simulink library "Vex_V5_Simulink_Expansion"  (R2022a)
settings: Solver=VariableStepAuto  StartTime=0.0  StopTime=10.0  RelTol=1e-3
libraries: $bdroot x48, vexv5lib x31, dspsigops x6, dsparch4 x2, slpidlib x1
(part 2 of 2)

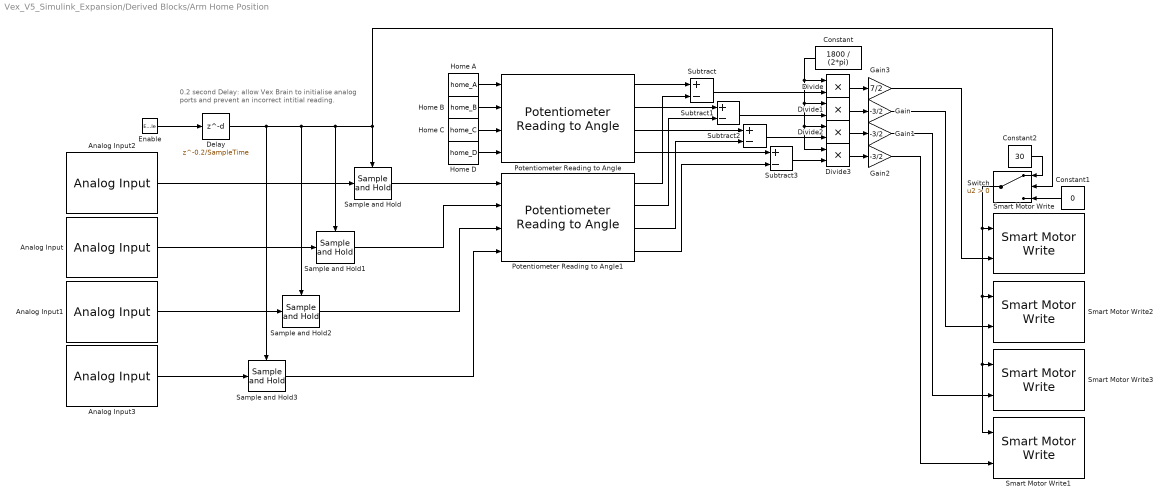
== system Vex_V5_Simulink_Expansion/Derived Blocks/Arm Home Position ==
  note: 0.2 second Delay: allow Vex Brain to initialise
      | analog ports and prevent an incorrect intitial reading.
  Enable : EnablePort  ShowOutputPort=on
  Analog Input : vexv5lib/Sensors/Analog Input  port=B  SampleTime=0.01
      settings: SourceProductBaseCode=VEXV5
  Analog Input1 : vexv5lib/Sensors/Analog Input  port=C  SampleTime=0.01
      settings: SourceProductBaseCode=VEXV5
  Analog Input2 : vexv5lib/Sensors/Analog Input  port=A  SampleTime=0.01
      settings: SourceProductBaseCode=VEXV5
  Analog Input3 : vexv5lib/Sensors/Analog Input  port=D  SampleTime=0.01
      settings: SourceProductBaseCode=VEXV5
  Constant : Constant  Value=1800 / (2*pi)
  Constant1 : Constant  Value=0
  Constant2 : Constant  Value=30
  Delay : Delay  DelayLength=0.2/SampleTime  SampleTime=SampleTime
  Divide{,1..3} (4 alike) : Product  Inputs=**
  Gain : Gain  Gain=-3/2
  Gain1 : Gain  Gain=-3/2
  Gain2 : Gain  Gain=-3/2
  Gain3 : Gain  Gain=7/2
  Home A : Constant  Value=home_A
  Home B : Constant  Value=home_B
  Home C : Constant  Value=home_C
  Home D : Constant  Value=home_D
  Potentiometer Reading to Angle : $bdroot/Unit Conversion/Potentiometer Reading to Angle  Home_A=home_A  Home_B=home_B  Home_C=home_C  Home_D=home_D
  Potentiometer Reading to Angle1 : $bdroot/Unit Conversion/Potentiometer Reading to Angle  Home_A=home_A  Home_B=home_B  Home_C=home_C  Home_D=home_D
  Sample and Hold{,1..3} (4 alike) : dspsigops/Sample and Hold  trig=Rising edge  initCond=0  latchinput=off
  Smart Motor Write : vexv5lib/Actuators/Smart Motor Write  motorPort=1  scaleFactor=18:1  MotorBrakeMode=Coast  OperationMode=Position Control
      settings: SourceProductBaseCode=VEXV5
  Smart Motor Write1 : vexv5lib/Actuators/Smart Motor Write  motorPort=4  scaleFactor=18:1  MotorBrakeMode=Coast  OperationMode=Position Control
      settings: SourceProductBaseCode=VEXV5
  Smart Motor Write2 : vexv5lib/Actuators/Smart Motor Write  motorPort=2  scaleFactor=18:1  MotorBrakeMode=Coast  OperationMode=Position Control
      settings: SourceProductBaseCode=VEXV5
  Smart Motor Write3 : vexv5lib/Actuators/Smart Motor Write  motorPort=3  scaleFactor=18:1  MotorBrakeMode=Coast  OperationMode=Position Control
      settings: SourceProductBaseCode=VEXV5
  Subtract{,1..3} (4 alike) : Sum  Inputs=+-
  Switch : Switch  Criteria=u2 > Threshold  SaturateOnIntegerOverflow=off  InputSameDT=off
  wires:
  Delay/1 -> Sample and Hold3/Trigger, Sample and Hold2/Trigger, Sample and Hold1/Trigger, Switch/2, Sample and Hold/Trigger
  Enable/1 -> Delay/1
  Potentiometer Reading to Angle/4 -> Subtract3/1
  Home C/1 -> Potentiometer Reading to Angle/3
  Gain3/1 -> Smart Motor Write/2
  Gain2/1 -> Smart Motor Write1/2
  Home A/1 -> Potentiometer Reading to Angle/1
  Divide3/1 -> Gain2/1
  Subtract2/1 -> Divide2/2
  Divide/1 -> Gain3/1
  Divide1/1 -> Gain/1
  Subtract/1 -> Divide/2
  Gain/1 -> Smart Motor Write2/2
  Constant1/1 -> Switch/3
  Switch/1 -> Smart Motor Write1/1, Smart Motor Write3/1, Smart Motor Write2/1, Smart Motor Write/1
  Constant2/1 -> Switch/1
  Analog Input1/1 -> Sample and Hold2/1
  Analog Input/1 -> Sample and Hold1/1
  Potentiometer Reading to Angle1/3 -> Subtract2/2
  Subtract1/1 -> Divide1/2
  Analog Input3/1 -> Sample and Hold3/1
  Potentiometer Reading to Angle1/4 -> Subtract3/2
  Gain1/1 -> Smart Motor Write3/2
  Potentiometer Reading to Angle/3 -> Subtract2/1
  Subtract3/1 -> Divide3/2
  Sample and Hold2/1 -> Potentiometer Reading to Angle1/3
  Divide2/1 -> Gain1/1
  Potentiometer Reading to Angle1/2 -> Subtract1/2
  Analog Input2/1 -> Sample and Hold/1
  Sample and Hold3/1 -> Potentiometer Reading to Angle1/4
  Potentiometer Reading to Angle/1 -> Subtract/1
  Constant/1 -> Divide3/1, Divide2/1, Divide1/1, Divide/1
  Sample and Hold/1 -> Potentiometer Reading to Angle1/1
  Potentiometer Reading to Angle/2 -> Subtract1/1
  Home D/1 -> Potentiometer Reading to Angle/4
  Potentiometer Reading to Angle1/1 -> Subtract/2
  Home B/1 -> Potentiometer Reading to Angle/2
  Sample and Hold1/1 -> Potentiometer Reading to Angle1/2

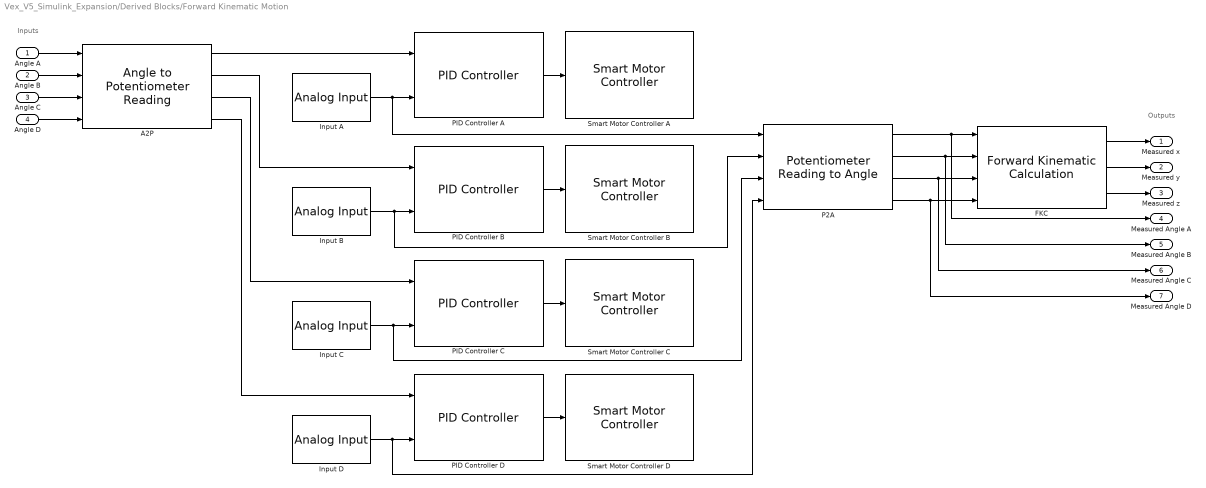
== system Vex_V5_Simulink_Expansion/Derived Blocks/Forward Kinematic Motion ==
  note: Inputs
  note: Outputs
  Angle A : Inport
  Angle B : Inport  Port=2
  Angle C : Inport  Port=3
  Angle D : Inport  Port=4
  A2P : $bdroot/Unit Conversion/Angle to Potentiometer Reading  Home_A=Home_A  Home_B=Home_B  Home_C=Home_C  Home_D=Home_D
  FKC : $bdroot/Core Blocks/Forward Kinematic Calculation
  Input A : vexv5lib/Sensors/Analog Input  port=A  SampleTime=SampleTime
      settings: SourceProductBaseCode=VEXV5
  Input B : vexv5lib/Sensors/Analog Input  port=B  SampleTime=SampleTime
      settings: SourceProductBaseCode=VEXV5
  Input C : vexv5lib/Sensors/Analog Input  port=C  SampleTime=SampleTime
      settings: SourceProductBaseCode=VEXV5
  Input D : vexv5lib/Sensors/Analog Input  port=D  SampleTime=SampleTime
      settings: SourceProductBaseCode=VEXV5
  P2A : $bdroot/Unit Conversion/Potentiometer Reading to Angle  Home_A=Home_A  Home_B=Home_B  Home_C=Home_C  Home_D=Home_D
  PID Controller A : $bdroot/Core Blocks/PID Controller  KP=KP_A  KI=KI_A  KD=KD_A  LimitOutput=off  limitHigh=limitHigh_A  limitLow=limitLow_A  AntiWindupMode=none  kb=kb_A
  PID Controller B : $bdroot/Core Blocks/PID Controller  KP=KP_B  KI=KI_B  KD=KD_B  LimitOutput=off  limitHigh=limitHigh_B  limitLow=limitLow_B  AntiWindupMode=none  kb=kb_B
  PID Controller C : $bdroot/Core Blocks/PID Controller  KP=KP_C  KI=KI_C  KD=KD_C  LimitOutput=off  limitHigh=limitHigh_C  limitLow=limitLow_C  AntiWindupMode=none  kb=kb_C
  PID Controller D : $bdroot/Core Blocks/PID Controller  KP=KP_D  KI=KI_D  KD=KD_D  LimitOutput=off  limitHigh=limitHigh_D  limitLow=limitLow_D  AntiWindupMode=none  kb=kb_D
  Smart Motor Controller A : $bdroot/Core Blocks/Smart Motor Controller  motorPort=1  OperationMode=Advanced Control  MotorBrakeMode=Coast
  Smart Motor Controller B : $bdroot/Core Blocks/Smart Motor Controller  motorPort=2  OperationMode=Advanced Control  MotorBrakeMode=Coast
  Smart Motor Controller C : $bdroot/Core Blocks/Smart Motor Controller  motorPort=3  OperationMode=Advanced Control  MotorBrakeMode=Coast
  Smart Motor Controller D : $bdroot/Core Blocks/Smart Motor Controller  motorPort=4  OperationMode=Advanced Control  MotorBrakeMode=Coast
  Measured x : Outport
  Measured y : Outport  Port=2
  Measured z : Outport  Port=3
  Measured Angle A : Outport  Port=4
  Measured Angle B : Outport  Port=5
  Measured Angle C : Outport  Port=6
  Measured Angle D : Outport  Port=7
  wires:
  A2P/3 -> PID Controller C/1
  PID Controller A/1 -> Smart Motor Controller A/1
  A2P/1 -> PID Controller A/1
  Input C/1 -> PID Controller C/2, P2A/3
  Angle D/1 -> A2P/4
  P2A/4 -> FKC/4, Measured Angle D/1
  P2A/3 -> FKC/3, Measured Angle C/1
  Angle C/1 -> A2P/3
  A2P/4 -> PID Controller D/1
  P2A/2 -> FKC/2, Measured Angle B/1
  FKC/1 -> Measured x/1
  Input B/1 -> PID Controller B/2, P2A/2
  P2A/1 -> FKC/1, Measured Angle A/1
  Input A/1 -> P2A/1, PID Controller A/2
  FKC/3 -> Measured z/1
  Input D/1 -> PID Controller D/2, P2A/4
  FKC/2 -> Measured y/1
  PID Controller B/1 -> Smart Motor Controller B/1
  PID Controller D/1 -> Smart Motor Controller D/1
  Angle A/1 -> A2P/1
  PID Controller C/1 -> Smart Motor Controller C/1
  A2P/2 -> PID Controller B/1
  Angle B/1 -> A2P/2

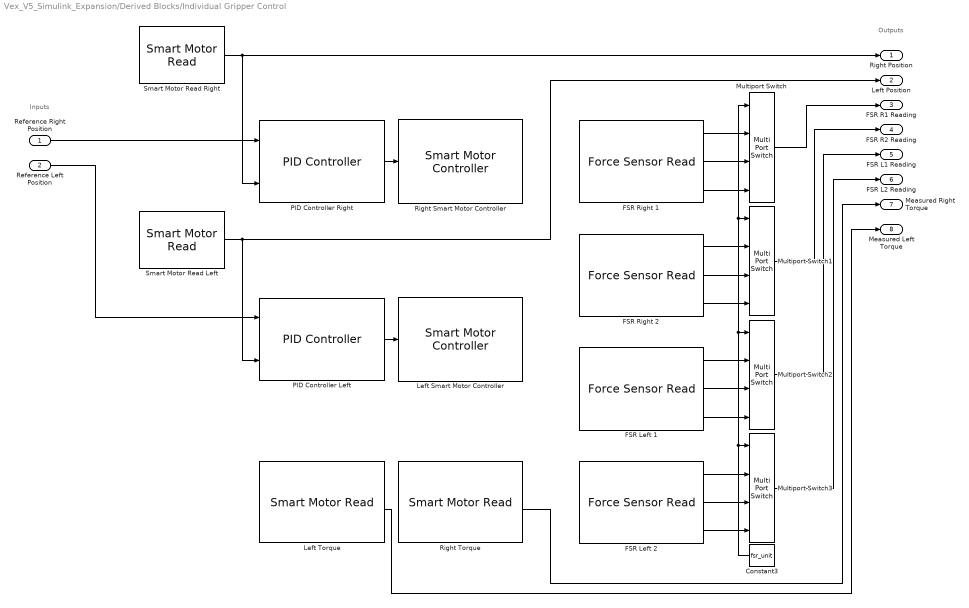
== system Vex_V5_Simulink_Expansion/Derived Blocks/Individual Gripper Control ==
  note: Outputs
  note: Inputs
  Reference Right Position : Inport
  Reference Left Position : Inport  Port=2
  Constant3 : Constant  Value=fsr_unit
  FSR Left 1 : $bdroot/Core Blocks/Force Sensor Read  port=A  SampleTime=SampleTime  Value=LA
  FSR Left 2 : $bdroot/Core Blocks/Force Sensor Read  port=B  SampleTime=SampleTime  Value=LB
  FSR Right 1 : $bdroot/Core Blocks/Force Sensor Read  port=D  SampleTime=SampleTime  Value=RA
  FSR Right 2 : $bdroot/Core Blocks/Force Sensor Read  port=C  SampleTime=SampleTime  Value=RB
  Left Smart Motor Controller : $bdroot/Core Blocks/Smart Motor Controller  motorPort=6  OperationMode=Advanced Control  MotorBrakeMode=Coast
  Left Torque : $bdroot/Core Blocks/Smart Motor Read  motorPort=6  SampleTime=SampleTime
  Multiport Switch{,1..3} (4 alike) : MultiPortSwitch  SaturateOnIntegerOverflow=off  InputSameDT=off
  PID Controller Left : $bdroot/Core Blocks/PID Controller  KP=KP  KI=KI  KD=KD  LimitOutput=off  limitHigh=limitHigh  limitLow=limitLow  AntiWindupMode=none  kb=kb
  PID Controller Right : $bdroot/Core Blocks/PID Controller  KP=KP  KI=KI  KD=KD  LimitOutput=off  limitHigh=limitHigh  limitLow=limitLow  AntiWindupMode=none  kb=kb
  Right Smart Motor Controller : $bdroot/Core Blocks/Smart Motor Controller  motorPort=3  OperationMode=Advanced Control  MotorBrakeMode=Coast
  Right Torque : $bdroot/Core Blocks/Smart Motor Read  motorPort=3  SampleTime=SampleTime
  Smart Motor Read Left : vexv5lib/Sensors/Smart Motor Read  motorPort=6  EncoderUnit=Degrees  resetOption=No reset  additionalOutput=off  SampleTime=SampleTime
      settings: SourceProductBaseCode=VEXV5
  Smart Motor Read Right : vexv5lib/Sensors/Smart Motor Read  motorPort=3  EncoderUnit=Degrees  resetOption=No reset  additionalOutput=off  SampleTime=SampleTime
      settings: SourceProductBaseCode=VEXV5
  Right Position : Outport
  Left Position : Outport  Port=2
  FSR R1 Reading : Outport  Port=3
  FSR R2 Reading : Outport  Port=4
  FSR L1 Reading : Outport  Port=5
  FSR L2 Reading : Outport  Port=6
  Measured Right Torque : Outport  Port=7
  Measured Left Torque : Outport  Port=8
  wires:
  Reference Right Position/1 -> PID Controller Right/1
  Reference Left Position/1 -> PID Controller Left/1
  FSR Right 1/1 -> Multiport Switch/2
  FSR Right 1/2 -> Multiport Switch/3
  FSR Right 1/3 -> Multiport Switch/4
  FSR Right 2/1 -> Multiport Switch1/2
  FSR Right 2/2 -> Multiport Switch1/3
  FSR Right 2/3 -> Multiport Switch1/4
  FSR Left 1/1 -> Multiport Switch2/2
  FSR Left 1/2 -> Multiport Switch2/3
  FSR Left 1/3 -> Multiport Switch2/4
  FSR Left 2/1 -> Multiport Switch3/2
  FSR Left 2/2 -> Multiport Switch3/3
  FSR Left 2/3 -> Multiport Switch3/4
  Multiport Switch/1 -> FSR R1 Reading/1
  Multiport Switch1/1 -> FSR R2 Reading/1
  Multiport Switch2/1 -> FSR L1 Reading/1
  Multiport Switch3/1 -> FSR L2 Reading/1
  Constant3/1 -> Multiport Switch/1, Multiport Switch1/1, Multiport Switch2/1, Multiport Switch3/1
  Smart Motor Read Right/1 -> Right Position/1, PID Controller Right/2
  Smart Motor Read Left/1 -> Left Position/1, PID Controller Left/2
  PID Controller Right/1 -> Right Smart Motor Controller/1
  PID Controller Left/1 -> Left Smart Motor Controller/1
  Right Torque/4 -> Measured Right Torque/1
  Left Torque/4 -> Measured Left Torque/1

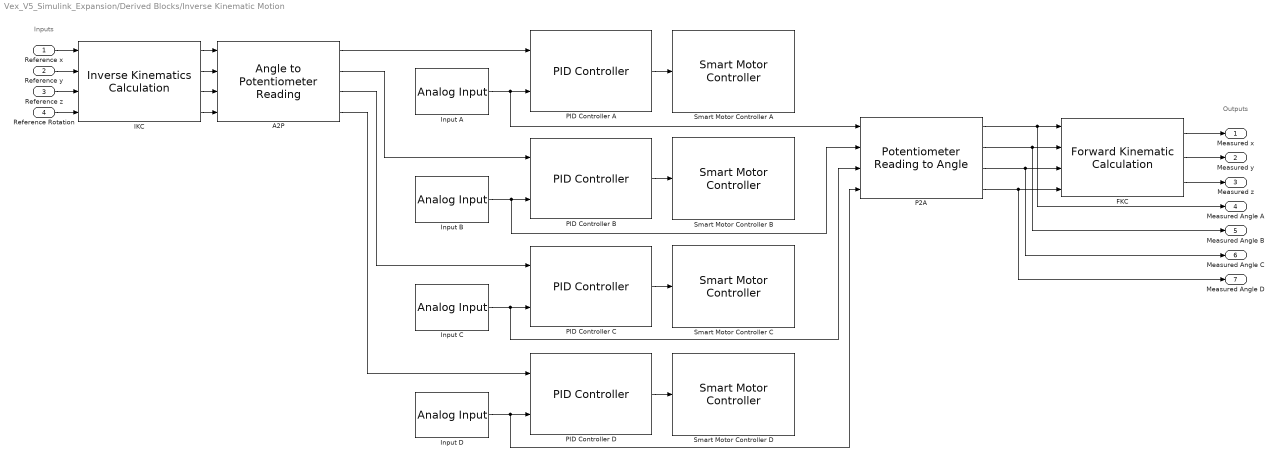
== system Vex_V5_Simulink_Expansion/Derived Blocks/Inverse Kinematic Motion ==
  note: Outputs
  note: Inputs
  Reference x : Inport
  Reference y : Inport  Port=2
  Reference z : Inport  Port=3
  Reference Rotation : Inport  Port=4
  A2P : $bdroot/Unit Conversion/Angle to Potentiometer Reading  Home_A=Home_A  Home_B=Home_B  Home_C=Home_C  Home_D=Home_D
  FKC : $bdroot/Core Blocks/Forward Kinematic Calculation
  IKC : $bdroot/Core Blocks/Inverse Kinematics Calculation
  Input A : vexv5lib/Sensors/Analog Input  port=A  SampleTime=0.01
      settings: SourceProductBaseCode=VEXV5
  Input B : vexv5lib/Sensors/Analog Input  port=B  SampleTime=0.01
      settings: SourceProductBaseCode=VEXV5
  Input C : vexv5lib/Sensors/Analog Input  port=C  SampleTime=0.01
      settings: SourceProductBaseCode=VEXV5
  Input D : vexv5lib/Sensors/Analog Input  port=D  SampleTime=0.01
      settings: SourceProductBaseCode=VEXV5
  P2A : $bdroot/Unit Conversion/Potentiometer Reading to Angle  Home_A=Home_A  Home_B=Home_B  Home_C=Home_C  Home_D=Home_D
  PID Controller A : $bdroot/Core Blocks/PID Controller  KP=KP_A  KI=KI_A  KD=KD_A  LimitOutput=off  limitHigh=limitHigh_A  limitLow=limitLow_A  AntiWindupMode=none  kb=kb_A
  PID Controller B : $bdroot/Core Blocks/PID Controller  KP=KP_B  KI=KI_B  KD=KD_B  LimitOutput=off  limitHigh=limitHigh_B  limitLow=limitLow_B  AntiWindupMode=none  kb=kb_B
  PID Controller C : $bdroot/Core Blocks/PID Controller  KP=KP_C  KI=KI_C  KD=KD_C  LimitOutput=off  limitHigh=limitHigh_C  limitLow=limitLow_C  AntiWindupMode=none  kb=kb_C
  PID Controller D : $bdroot/Core Blocks/PID Controller  KP=KP_D  KI=KI_D  KD=KD_D  LimitOutput=off  limitHigh=limitHigh_D  limitLow=limitLow_D  AntiWindupMode=none  kb=kb_D
  Smart Motor Controller A : $bdroot/Core Blocks/Smart Motor Controller  motorPort=1  OperationMode=Advanced Control  MotorBrakeMode=Coast
  Smart Motor Controller B : $bdroot/Core Blocks/Smart Motor Controller  motorPort=2  OperationMode=Advanced Control  MotorBrakeMode=Coast
  Smart Motor Controller C : $bdroot/Core Blocks/Smart Motor Controller  motorPort=3  OperationMode=Advanced Control  MotorBrakeMode=Coast
  Smart Motor Controller D : $bdroot/Core Blocks/Smart Motor Controller  motorPort=4  OperationMode=Advanced Control  MotorBrakeMode=Coast
  Measured x : Outport
  Measured y : Outport  Port=2
  Measured z : Outport  Port=3
  Measured Angle A : Outport  Port=4
  Measured Angle B : Outport  Port=5
  Measured Angle C : Outport  Port=6
  Measured Angle D : Outport  Port=7
  wires:
  A2P/2 -> PID Controller B/1
  FKC/2 -> Measured y/1
  Input C/1 -> PID Controller C/2, P2A/3
  PID Controller C/1 -> Smart Motor Controller C/1
  Input A/1 -> P2A/1, PID Controller A/2
  PID Controller A/1 -> Smart Motor Controller A/1
  PID Controller B/1 -> Smart Motor Controller B/1
  PID Controller D/1 -> Smart Motor Controller D/1
  FKC/3 -> Measured z/1
  P2A/1 -> FKC/1, Measured Angle A/1
  A2P/1 -> PID Controller A/1
  A2P/4 -> PID Controller D/1
  Input B/1 -> PID Controller B/2, P2A/2
  P2A/3 -> FKC/3, Measured Angle C/1
  Input D/1 -> PID Controller D/2, P2A/4
  FKC/1 -> Measured x/1
  P2A/2 -> FKC/2, Measured Angle B/1
  P2A/4 -> FKC/4, Measured Angle D/1
  IKC/1 -> A2P/1
  IKC/2 -> A2P/2
  IKC/3 -> A2P/3
  IKC/4 -> A2P/4
  Reference x/1 -> IKC/1
  Reference y/1 -> IKC/2
  Reference z/1 -> IKC/3
  Reference Rotation/1 -> IKC/4
  A2P/3 -> PID Controller C/1

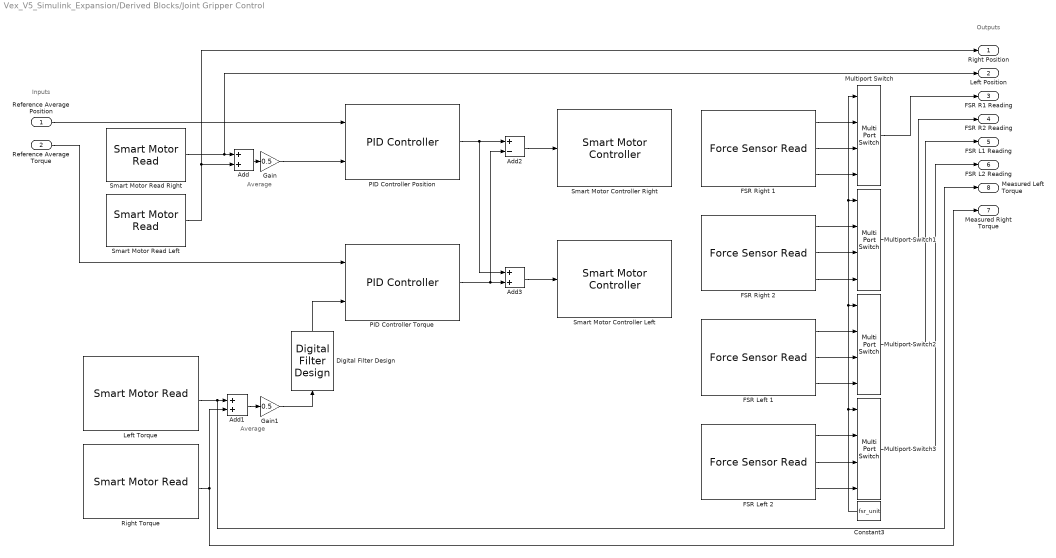
== system Vex_V5_Simulink_Expansion/Derived Blocks/Joint Gripper Control ==
  note: Average
  note: Inputs
  note: Outputs
  note: Average
  Reference Average Position : Inport
  Reference Average Torque : Inport  Port=2
  Add : Sum
  Add1 : Sum
  Add2 : Sum  Inputs=+-
  Add3 : Sum
  Constant3 : Constant  Value=fsr_unit
  Digital Filter Design : dsparch4/Digital Filter Design  mwdsp_browser_bugfix_var=off
  FSR Left 1 : $bdroot/Core Blocks/Force Sensor Read  port=H  SampleTime=SampleTime  Value=LA
  FSR Left 2 : $bdroot/Core Blocks/Force Sensor Read  port=G  SampleTime=SampleTime  Value=LB
  FSR Right 1 : $bdroot/Core Blocks/Force Sensor Read  port=F  SampleTime=SampleTime  Value=RA
  FSR Right 2 : $bdroot/Core Blocks/Force Sensor Read  port=E  SampleTime=SampleTime  Value=RB
  Gain : Gain  Gain=0.5
  Gain1 : Gain  Gain=0.5
  Left Torque : $bdroot/Core Blocks/Smart Motor Read  motorPort=5  SampleTime=SampleTime
  Multiport Switch{,1..3} (4 alike) : MultiPortSwitch  SaturateOnIntegerOverflow=off  InputSameDT=off
  PID Controller Position : $bdroot/Core Blocks/PID Controller  KP=KP_position  KI=KI_positon  KD=KD_position  LimitOutput=off  limitHigh=limitHigh_position  limitLow=limitLow_position  AntiWindupMode=none  kb=kb_position
  PID Controller Torque : $bdroot/Core Blocks/PID Controller  KP=KP  KI=KI  KD=KD  LimitOutput=off  limitHigh=limitHigh  limitLow=limitLow  AntiWindupMode=none  kb=kb
  Right Torque : $bdroot/Core Blocks/Smart Motor Read  motorPort=6  SampleTime=SampleTime
  Smart Motor Controller Left : $bdroot/Core Blocks/Smart Motor Controller  motorPort=5  OperationMode=Advanced Control  MotorBrakeMode=Coast
  Smart Motor Controller Right : $bdroot/Core Blocks/Smart Motor Controller  motorPort=6  OperationMode=Advanced Control  MotorBrakeMode=Coast
  Smart Motor Read Left : vexv5lib/Sensors/Smart Motor Read  motorPort=5  EncoderUnit=Degrees  resetOption=No reset  additionalOutput=off  SampleTime=SampleTime
      settings: SourceProductBaseCode=VEXV5
  Smart Motor Read Right : vexv5lib/Sensors/Smart Motor Read  motorPort=6  EncoderUnit=Degrees  resetOption=No reset  additionalOutput=off  SampleTime=SampleTime
      settings: SourceProductBaseCode=VEXV5
  Right Position : Outport
  Left Position : Outport  Port=2
  FSR R1 Reading : Outport  Port=3
  FSR R2 Reading : Outport  Port=4
  FSR L1 Reading : Outport  Port=5
  FSR L2 Reading : Outport  Port=6
  Measured Right Torque : Outport  Port=7
  Measured Left Torque : Outport  Port=8
  wires:
  FSR Right 2/1 -> Multiport Switch1/2
  FSR Right 2/3 -> Multiport Switch1/4
  FSR Left 1/1 -> Multiport Switch2/2
  FSR Right 1/2 -> Multiport Switch/3
  Reference Average Torque/1 -> PID Controller Torque/1
  Constant3/1 -> Multiport Switch/1, Multiport Switch1/1, Multiport Switch2/1, Multiport Switch3/1
  Multiport Switch3/1 -> FSR L2 Reading/1
  FSR Left 1/2 -> Multiport Switch2/3
  FSR Left 2/3 -> Multiport Switch3/4
  FSR Right 2/2 -> Multiport Switch1/3
  Multiport Switch1/1 -> FSR R2 Reading/1
  FSR Right 1/3 -> Multiport Switch/4
  FSR Left 2/1 -> Multiport Switch3/2
  FSR Left 2/2 -> Multiport Switch3/3
  Multiport Switch/1 -> FSR R1 Reading/1
  FSR Right 1/1 -> Multiport Switch/2
  Multiport Switch2/1 -> FSR L1 Reading/1
  FSR Left 1/3 -> Multiport Switch2/4
  Reference Average Position/1 -> PID Controller Position/1
  Smart Motor Read Right/1 -> Left Position/1, Add/1
  Smart Motor Read Left/1 -> Add/2, Right Position/1
  Add/1 -> Gain/1
  Gain/1 -> PID Controller Position/2
  Add1/1 -> Gain1/1
  Left Torque/4 -> Measured Left Torque/1, Add1/1
  Right Torque/4 -> Measured Right Torque/1, Add1/2
  PID Controller Torque/1 -> Add2/2, Add3/2
  Gain1/1 -> Digital Filter Design/1
  PID Controller Position/1 -> Add3/1, Add2/1
  Add2/1 -> Smart Motor Controller Right/1
  Add3/1 -> Smart Motor Controller Left/1
  Digital Filter Design/1 -> PID Controller Torque/2

== system Vex_V5_Simulink_Expansion/Derived Blocks/Motor Torque Control ==
  note: Outputs
  note: Inputs
  Reference Torque : Inport
  Digital Filter Design : dsparch4/Digital Filter Design  mwdsp_browser_bugfix_var=off
  Motor Read : $bdroot/Core Blocks/Smart Motor Read  motorPort=5  SampleTime=SampleTime
  PID : $bdroot/Core Blocks/PID Controller  KP=KP  KI=KI  KD=KD  LimitOutput=off  limitHigh=limitHigh  limitLow=limitLow  AntiWindupMode=none  kb=kb
  Smart Motor Controller : $bdroot/Core Blocks/Smart Motor Controller  motorPort=5  OperationMode=Advanced Control  MotorBrakeMode=Coast
  Measured Torque : Outport
  Measured Voltage : Outport  Port=2
  Measured Current : Outport  Port=3
  wires:
  Reference Torque/1 -> PID/1
  PID/1 -> Smart Motor Controller/1
  Motor Read/1 -> Measured Voltage/1
  Motor Read/2 -> Measured Current/1
  Motor Read/4 -> Digital Filter Design/1
  Digital Filter Design/1 -> PID/2, Measured Torque/1

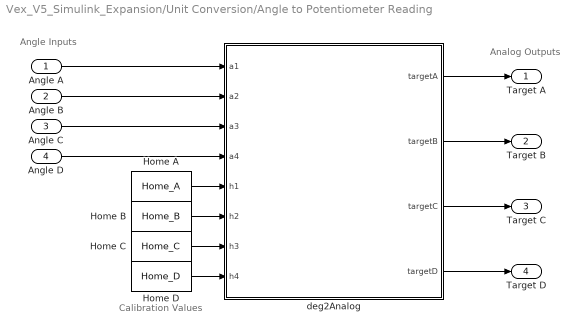
== system Vex_V5_Simulink_Expansion/Unit Conversion/Angle to Potentiometer Reading ==
  note: Calibration Values
  note: Angle Inputs
  note: Analog Outputs
  Angle A : Inport
  Angle B : Inport  Port=2
  Angle C : Inport  Port=3
  Angle D : Inport  Port=4
  Home A : Constant  Value=Home_A
  Home B : Constant  Value=Home_B
  Home C : Constant  Value=Home_C
  Home D : Constant  Value=Home_D
  deg2Analog : MATLAB Function  TreatAsAtomicUnit=on
  Target A : Outport
  Target B : Outport  Port=2
  Target C : Outport  Port=3
  Target D : Outport  Port=4
  wires:
  Home A/1 -> deg2Analog/5(h1)
  Home B/1 -> deg2Analog/6(h2)
  Home C/1 -> deg2Analog/7(h3)
  Home D/1 -> deg2Analog/8(h4)
  Angle D/1 -> deg2Analog/4(a4)
  Angle C/1 -> deg2Analog/3(a3)
  Angle B/1 -> deg2Analog/2(a2)
  Angle A/1 -> deg2Analog/1(a1)
  deg2Analog/1(targetA) -> Target A/1
  deg2Analog/2(targetB) -> Target B/1
  deg2Analog/3(targetC) -> Target C/1
  deg2Analog/4(targetD) -> Target D/1

== system Vex_V5_Simulink_Expansion/Unit Conversion/Force to Resistance ==
  note: Input
  note: Output
  Force : Inport
  Constant : Constant  Value=K
  Constant1 : Constant
  Divide : Product  Inputs=*/
  Divide1 : Product  Inputs=*/
  Gradient : Constant  Value=m
  Power : Math  Operator=pow
  Resistance : Outport
  wires:
  Power/1 -> Resistance/1
  Force/1 -> Divide/1
  Constant/1 -> Divide/2
  Gradient/1 -> Divide1/2
  Constant1/1 -> Divide1/1
  Divide/1 -> Power/1
  Divide1/1 -> Power/2

== system Vex_V5_Simulink_Expansion/Unit Conversion/Joint to Motor Angle ==
  note: Outputs
  note: Inputs
  Joint Angle A : Inport
  Joint Angle B : Inport  Port=2
  Joint Angle C : Inport  Port=3
  Joint Angle D : Inport  Port=4
  jointToMotor : MATLAB Function  TreatAsAtomicUnit=on
  Motor Angle A : Outport
  Motor Angle B : Outport  Port=2
  Motor Angle C : Outport  Port=3
  Motor Angle D : Outport  Port=4
  wires:
  jointToMotor/1(motorA) -> Motor Angle A/1
  jointToMotor/2(motorB) -> Motor Angle B/1
  jointToMotor/3(motorC) -> Motor Angle C/1
  jointToMotor/4(motorD) -> Motor Angle D/1
  Joint Angle D/1 -> jointToMotor/4(jointD)
  Joint Angle C/1 -> jointToMotor/3(jointC)
  Joint Angle B/1 -> jointToMotor/2(jointB)
  Joint Angle A/1 -> jointToMotor/1(jointA)

== system Vex_V5_Simulink_Expansion/Unit Conversion/Motor to Joint Angle ==
  note: Inputs
  note: Outputs
  Motor Angle A : Inport
  Motor Angle B : Inport  Port=2
  Motor Angle C : Inport  Port=3
  Motor Angle D : Inport  Port=4
  motorToJoint : MATLAB Function  TreatAsAtomicUnit=on
  Joint Angle A : Outport
  Joint Angle B : Outport  Port=2
  Joint Angle C : Outport  Port=3
  Joint Angle D : Outport  Port=4
  wires:
  Motor Angle A/1 -> motorToJoint/1(motorA)
  Motor Angle B/1 -> motorToJoint/2(motorB)
  Motor Angle C/1 -> motorToJoint/3(motorC)
  Motor Angle D/1 -> motorToJoint/4(motorD)
  motorToJoint/4(jointD) -> Joint Angle D/1
  motorToJoint/3(jointC) -> Joint Angle C/1
  motorToJoint/2(jointB) -> Joint Angle B/1
  motorToJoint/1(jointA) -> Joint Angle A/1

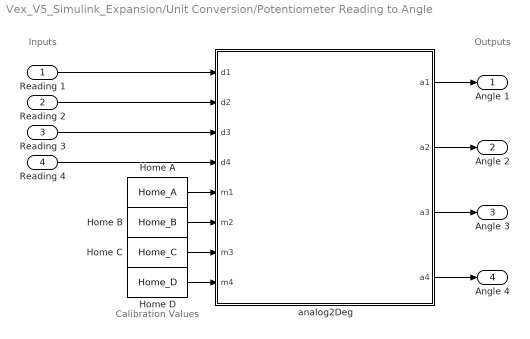
== system Vex_V5_Simulink_Expansion/Unit Conversion/Potentiometer Reading to Angle ==
  note: Outputs
  note: Inputs
  note: Calibration Values
  Reading 1 : Inport
  Reading 2 : Inport  Port=2
  Reading 3 : Inport  Port=3
  Reading 4 : Inport  Port=4
  Home A : Constant  Value=Home_A
  Home B : Constant  Value=Home_B
  Home C : Constant  Value=Home_C
  Home D : Constant  Value=Home_D
  analog2Deg : MATLAB Function  TreatAsAtomicUnit=on
  Angle 1 : Outport
  Angle 2 : Outport  Port=2
  Angle 3 : Outport  Port=3
  Angle 4 : Outport  Port=4
  wires:
  analog2Deg/1(a1) -> Angle 1/1
  analog2Deg/2(a2) -> Angle 2/1
  analog2Deg/3(a3) -> Angle 3/1
  analog2Deg/4(a4) -> Angle 4/1
  Reading 1/1 -> analog2Deg/1(d1)
  Reading 2/1 -> analog2Deg/2(d2)
  Reading 3/1 -> analog2Deg/3(d3)
  Reading 4/1 -> analog2Deg/4(d4)
  Home A/1 -> analog2Deg/5(m1)
  Home B/1 -> analog2Deg/6(m2)
  Home C/1 -> analog2Deg/7(m3)
  Home D/1 -> analog2Deg/8(m4)

== system Vex_V5_Simulink_Expansion/Unit Conversion/Resistance to Force ==
  note: Output
  note: Input
  Resistance : Inport
  Constant : Constant  Value=K
  Divide : Product  Inputs=**
  Gradient : Constant  Value=m
  Power : Math  Operator=pow
  Force : Outport
  wires:
  Gradient/1 -> Power/2
  Power/1 -> Divide/2
  Constant/1 -> Divide/1
  Resistance/1 -> Power/1
  Divide/1 -> Force/1

== system Vex_V5_Simulink_Expansion/Unit Conversion/deg2Rad ==
  Input : Inport
  Constant : Constant  Value=pi
  Constant1 : Constant  Value=180
  Divide : Product  Inputs=**/
  Output : Outport
  wires:
  Input/1 -> Divide/2
  Divide/1 -> Output/1
  Constant/1 -> Divide/1
  Constant1/1 -> Divide/3

== system Vex_V5_Simulink_Expansion/Unit Conversion/rad2Deg ==
  Input : Inport
  Constant : Constant  Value=180
  Constant1 : Constant  Value=pi
  Divide : Product  Inputs=**/
  Output : Outport
  wires:
  Constant1/1 -> Divide/3
  Constant/1 -> Divide/1
  Divide/1 -> Output/1
  Input/1 -> Divide/2

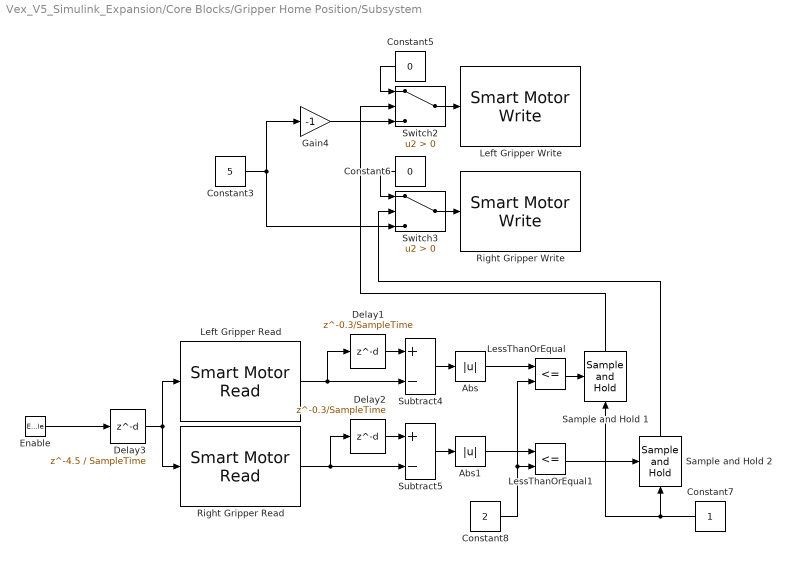
== system Vex_V5_Simulink_Expansion/Core Blocks/Gripper Home Position/Subsystem ==
  Enable : EnablePort  ShowOutputPort=on
  Abs : Abs  SaturateOnIntegerOverflow=off
  Abs1 : Abs  SaturateOnIntegerOverflow=off
  Constant3 : Constant  Value=5
  Constant5 : Constant  Value=0
  Constant6 : Constant  Value=0
  Constant7 : Constant
  Constant8 : Constant  Value=2
  Delay1 : Delay  DelayLength=0.3/SampleTime  SampleTime=SampleTime
  Delay2 : Delay  DelayLength=0.3/SampleTime  SampleTime=SampleTime
  Delay3 : Delay  DelayLength=4.5 / SampleTime  SampleTime=SampleTime
  Gain4 : Gain  Gain=-1
  Left Gripper Read : vexv5lib/Sensors/Smart Motor Read  motorPort=5  EncoderUnit=Degrees  resetOption=Reset by external signal  additionalOutput=off  SampleTime=SampleTime
      settings: SourceProductBaseCode=VEXV5
  Left Gripper Write : vexv5lib/Actuators/Smart Motor Write  motorPort=5  scaleFactor=18:1  MotorBrakeMode=Coast  OperationMode=Velocity Control
      settings: SourceProductBaseCode=VEXV5
  LessThanOrEqual : RelationalOperator  Operator=<=  OutDataTypeStr=boolean  RndMeth=Simplest  InputSameDT=off
  LessThanOrEqual1 : RelationalOperator  Operator=<=  OutDataTypeStr=boolean  RndMeth=Simplest  InputSameDT=off
  Right Gripper Read : vexv5lib/Sensors/Smart Motor Read  motorPort=6  EncoderUnit=Degrees  resetOption=Reset by external signal  additionalOutput=off  SampleTime=SampleTime
      settings: SourceProductBaseCode=VEXV5
  Right Gripper Write : vexv5lib/Actuators/Smart Motor Write  motorPort=6  scaleFactor=18:1  MotorBrakeMode=Coast  OperationMode=Velocity Control
      settings: SourceProductBaseCode=VEXV5
  Sample and Hold 1 : dspsigops/Sample and Hold  trig=Rising edge  initCond=0  latchinput=off
  Sample and Hold 2 : dspsigops/Sample and Hold  trig=Rising edge  initCond=0  latchinput=off
  Subtract4 : Sum  Inputs=+-
  Subtract5 : Sum  Inputs=+-
  Switch2 : Switch  Criteria=u2 > Threshold  SaturateOnIntegerOverflow=off  InputSameDT=off
  Switch3 : Switch  Criteria=u2 > Threshold  SaturateOnIntegerOverflow=off  InputSameDT=off
  wires:
  Switch2/1 -> Left Gripper Write/1
  Constant8/1 -> LessThanOrEqual/2, LessThanOrEqual1/2
  Constant6/1 -> Switch3/1
  Constant7/1 -> Sample and Hold 1/1, Sample and Hold 2/1
  Subtract4/1 -> Abs/1
  Constant5/1 -> Switch2/1
  Delay3/1 -> Left Gripper Read/1, Right Gripper Read/1
  Left Gripper Read/1 -> Delay1/1, Subtract4/2
  Switch3/1 -> Right Gripper Write/1
  LessThanOrEqual/1 -> Sample and Hold 1/Trigger
  Gain4/1 -> Switch2/3
  Right Gripper Read/1 -> Delay2/1, Subtract5/2
  Abs1/1 -> LessThanOrEqual1/1
  Constant3/1 -> Gain4/1, Switch3/3
  Delay2/1 -> Subtract5/1
  Sample and Hold 1/1 -> Switch2/2
  LessThanOrEqual1/1 -> Sample and Hold 2/Trigger
  Abs/1 -> LessThanOrEqual/1
  Enable/1 -> Delay3/1
  Delay1/1 -> Subtract4/1
  Subtract5/1 -> Abs1/1
  Sample and Hold 2/1 -> Switch3/2

== stateflow chart Vex_V5_Simulink_Expansion/Core Blocks/Initialisation Routine/Initialisation Schedule ==
  state Homing
    enable_homing = 1;
    enable_user = 0;
  state User
    enable_homing = 0;
    enable_user = 1;
  (default) -> Homing
  Homing -> User : [simulation_time > 5]
  data: simulation_time input; enable_homing output; enable_user output

== matlab function Vex_V5_Simulink_Expansion/Unit Conversion/Potentiometer Reading to Angle/analog2Deg ==
  data: d1 input; d2 input; d3 input; d4 input; a1 output; m1 input; m2 input; m3 input; m4 input; a2 output; a3 output; a4 output
function [a1,a2,a3,a4] = analog2Deg(d1,d2,d3,d4,m1,m2,m3,m4)
    
    % Vex Brain has a 10 bit ADC == 4096 resolution
    % Potentiometer has 333 degrees of rotation
    scale = ((4096 / 333)*360) / (2*pi);

    % Home angles
    conv = 2*pi / 360;
    ang1 = 0;
    ang2 = 20*conv;
    ang3 = 3.07*conv;
    ang4 = 93.07*conv;

    % Find angles relative to home position
    t1 = (d1 - m1) / scale;
    t2 = (m2 - d2) / (3*scale);
    t3 = (m3 - d3) / (3*scale);
    t4 = (m4 - d4) / (3*scale);

    % Compute actual motor angles
    a1 = t1 + ang1;
    a2 = t2 + ang2;
    a3 = t3 + ang3;
    a4 = t4 + ang4;

== matlab function Vex_V5_Simulink_Expansion/Core Blocks/Force Sensor Read/MATLAB Function ==
  data: volIn input; volOut input; res input; forceRes output
function forceRes = invPD(volIn,volOut,res)
    forceRes = (volIn / volOut)*res - res;

== matlab function Vex_V5_Simulink_Expansion/Core Blocks/Inverse Kinematics Calculation/MATLAB Function ==
  data: x input; a1 output; y input; z input; rotation input; a2 output; a3 output; a4 output
function [a1,a2,a3,a4]= inverseKinematics(x,y,z,rotation)

    % Geometric constants
    conv = 25.4;
    L_1 = 7*conv;
    L_2 = 7*conv;
    L_3 = 2*conv;
    AR = 0.7224*conv;
    AZ = (5.296+1.375)*conv;

    % Handle end effector position/rotation
    x_adj = x - L_3*sin(rotation)*cos(atan(y/x));
    y_adj = y - L_3*sin(rotation)*sin(atan(y/x));
    z_adj = z - L_3*cos(rotation);
    t4 = rotation;

    % Fix base angle to reduce unknowns
    t1 = atan(y_adj/x_adj);
    XE = sqrt(x_adj^2 + y_adj^2) - AR;
    YE = z_adj - AZ;
    
    % Derived using Matlab Symbolic Maths
    t2 = 2*atan((2*L_1*XE - (- L_1^4 + 2*L_1^2*L_2^2 + 2*L_1^2*XE^2 + ...
        2*L_1^2*YE^2 - L_2^4 + 2*L_2^2*XE^2 + 2*L_2^2*YE^2 - XE^4 - ...
        2*XE^2*YE^2 - YE^4)^(1/2))/(L_1^2 + 2*L_1*YE - L_2^2 + XE^2 + YE^2));
    
    % As above
    t3 = 2*atan((2*L_2*XE - ((- L_1^2 + 2*L_1*L_2 - L_2^2 + XE^2 + YE^2) ...
        *(L_1^2 + 2*L_1*L_2 + L_2^2 - XE^2 - YE^2))^(1/2))/ ...
        (- L_1^2 + L_2^2 - 2*L_2*YE + XE^2 + YE^2));

    % Above formulas can produce complex results, the following fixes that
    a1 = NaN(size(t1));
    a2 = NaN(size(t2));
    a3 = NaN(size(t3));
    a4 = NaN(size(t4));

    tf_mat = imag(t1) == 0;
    a1(tf_mat) = real(t1(tf_mat));

    tf_mat = imag(t2) == 0;
    a2(tf_mat) = real(t2(tf_mat));

    tf_mat = imag(t3) == 0;
    a3(tf_mat) = real(t3(tf_mat));

    tf_mat = imag(t4) == 0;
    a4(tf_mat) = real(t4(tf_mat));

== matlab function Vex_V5_Simulink_Expansion/Unit Conversion/Motor to Joint Angle/motorToJoint ==
  data: motorA input; jointA output; motorB input; motorC input; motorD input; jointB output; jointC output; jointD output
function [jointA,jointB,jointC,jointD] = motorToArm(motorA,motorB,motorC,motorD)
    
    % Joints A and B are the same in both reference frames
    jointA = motorA;
    jointB = motorB;
    % Joints C and D have angles dependant on previous members
    jointC = pi - (motorB + motorC);
    jointD = 3*pi - (pi + motorC + motorD);

== matlab function Vex_V5_Simulink_Expansion/Unit Conversion/Joint to Motor Angle/jointToMotor ==
  data: jointA input; motorA output; jointB input; jointC input; jointD input; motorB output; motorC output; motorD output
function [motorA,motorB,motorC,motorD] = jointToMotor(jointA,jointB,jointC,jointD)
    
    % Joints A and B are the same in both reference frames
    motorA = jointA;
    motorB = jointB;
    % Joints C and D have angles dependant on previous members
    motorC = pi - (jointB + jointC);
    motorD = pi - jointD + jointC + jointB;

== matlab function Vex_V5_Simulink_Expansion/Core Blocks/Forward Kinematic Calculation/MATLAB Function5 ==
  data: x output; a1 input; y output; a2 input; a3 input; a4 input; z output
function [x,y,z] = forward_kinematics(a1, a2, a3, a4)

    % Define geometric constants
    conv = 25.4;        % Convert from inches to mm
    AR = 0.7224*conv;
    AZ = (5.296+1.375)*conv;
    BC = 7*conv;
    CD = 7*conv;
    DE = 2*conv;

    % Implement derived forward dynamics equations
    x = (AR + BC*sin(a2) + CD*sin(a3) + DE*sin(a4))*cos(a1);
    y = (AR + BC*sin(a2) + CD*sin(a3) + DE*sin(a4))*sin(a1);
    z = (AZ + BC*cos(a2) - CD*cos(a3) + DE*cos(a4));

== matlab function Vex_V5_Simulink_Expansion/Unit Conversion/Angle to Potentiometer Reading/deg2Analog ==
  data: a1 input; a2 input; a3 input; a4 input; targetA output; h1 input; h2 input; h3 input; h4 input; targetB output; targetC output; targetD output
function [targetA,targetB,targetC,targetD] = deg2Analog(a1,a2,a3,a4,h1,h2,h3,h4)
    
    % Vex Brain has a 10 bit ADC == 4096 resolution
    % Potentiometer has 333 degrees of rotation
    scale = ((4096 / 333)*360) / (2*pi);

    % Home angles
    conv = 2*pi / 360;
    ang1 = 0;
    ang2 = 20*conv;
    ang3 = 3.07*conv;
    ang4 = 93.07*conv;

    % Subtract home angles from desired position
    t1 = a1 - ang1;
    t2 = a2 - ang2;
    t3 = a3 - ang3;
    t4 = a4 - ang4;

    % Scale angles, including gear ratios
    targetA = h1 + t1*scale;
    targetB = h2 - t2*scale*3;
    targetC = h3 - t3*scale*3;
    targetD = h4 - t4*scale*3;
